simulink model "modem"  (R2019b)
settings: Solver=VariableStepAuto  StartTime=0.0  StopTime=1  RelTol=1e-3
libraries: commsink2 x1
settings Model: Creator=kaushik  LastModifiedBy=kaushik
settings DataIOCC: ReturnWorkspaceOutputs=off
settings OptimizationCC: BlockReduction=off  ConditionallyExecuteInputs=off
settings DebuggingCC: InheritedTsInSrcMsg=none

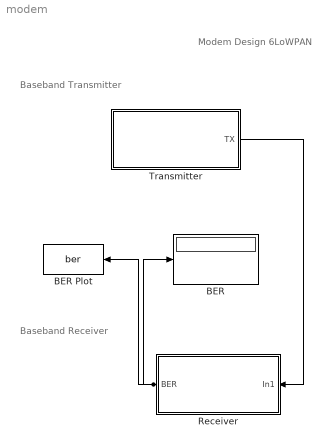
== system modem ==
  note: Baseband Transmitter
  note: Modem Design 6LoWPAN
  note: Baseband Receiver
  "BER " : Display
  BER Plot : ToWorkspace  VariableName=ber  SampleTime=-1
      settings: MaxDataPoints=2  Save2DSignal=2-D array (concatenate along first dimension)
  Receiver : Subsystem
      mask Display: disp('IEEE 802.15\nReceiver')
  Transmitter : Subsystem
  wires:
  Transmitter/1(TX) -> Receiver/1(In1)
  Receiver/1(BER) -> "BER "/1, BER Plot/1

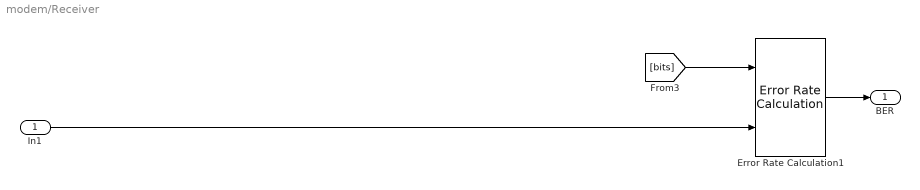
== system modem/Receiver ==
  In1 : Inport
  Error Rate Calculation1 : commsink2/Error Rate Calculation  N=4  st_delay=0  cp_mode=Entire frame  subframe=[]  PMode=Port  WsName=ErrorVec  RsMode2=off  stop=on  numErr=100  maxBits=1e7
      settings: SourceProductName=Communications Toolbox
  BER : Outport  VectorParamsAs1DForOutWhenUnconnected=off
  wires:
  In1/1 -> Error Rate Calculation1/2
  [bits] -> Error Rate Calculation1/1
  Error Rate Calculation1/1 -> BER/1

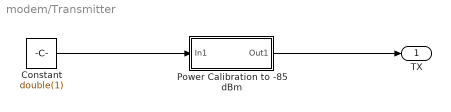
== system modem/Transmitter ==
  Constant : Constant  Value=double(1)  OutDataTypeStr=double  SampleTime=-1
  Power Calibration to -85 dBm : Subsystem  mask(dB Gain){dB=double(-118.159), intype=Amplitude}
      mask prompts: dB "Gain, dB:"; intype "Input signal:"
      mask help: Apply a gain specified in dB.
      mask Help: eval('blocksethelp');
      mask TypeOptions intype: Power | Amplitude
      mask Display: fprintf(s)
  TX : Outport
  wires:
  Constant/1 -> Power Calibration to -85 dBm/1(In1)
  Power Calibration to -85 dBm/1(Out1) -> TX/1

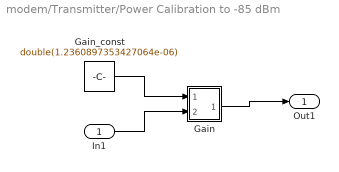
== system modem/Transmitter/Power Calibration to -85 dBm ==
  In1 : Inport  OutDataTypeStr=double  SampleTime=10
  Gain : Subsystem
      mask Display: disp('NFP\nmul');
  Gain_const : Constant  Value=double(1.2360897353427064e-06)  OutDataTypeStr=double  SampleTime=-1
  Out1 : Outport
  wires:
  Gain_const/1 -> Gain/1(In1)
  Gain/1(Out1) -> Out1/1
  In1/1 -> Gain/2(In2)

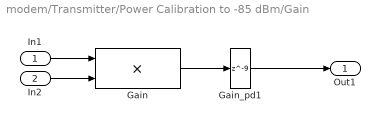
== system modem/Transmitter/Power Calibration to -85 dBm/Gain ==
  In1 : Inport
  In2 : Inport  Port=2
  Gain : Product  Inputs=**  OutDataTypeStr=double  SampleTime=10
  Gain_pd1 : Delay  DelayLength=9
  Out1 : Outport
  wires:
  In1/1 -> Gain/1
  In2/1 -> Gain/2
  Gain/1 -> Gain_pd1/1
  Gain_pd1/1 -> Out1/1
